simulink model "CubeSat"  (R2024b)
settings: Solver=VariableStepAuto  StartTime=0.0  StopTime=10.0  RelTol=1e-3
undefined symbols (not defined in the file or in its folder): act, env, flag, IC, orb, sat, sens
libraries: matrix_library x14, simulink_extras x2
(part 1 of 3)
settings Model: Creator=filippocamaleonte  LastModifiedBy=filippocamaleonte

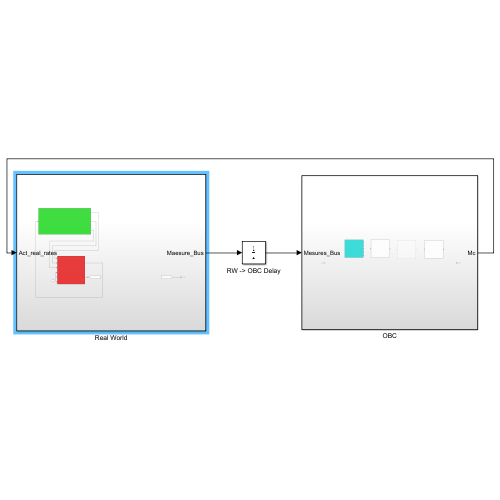
[thumbnail: Simulink's stored preview of the top-level diagram]
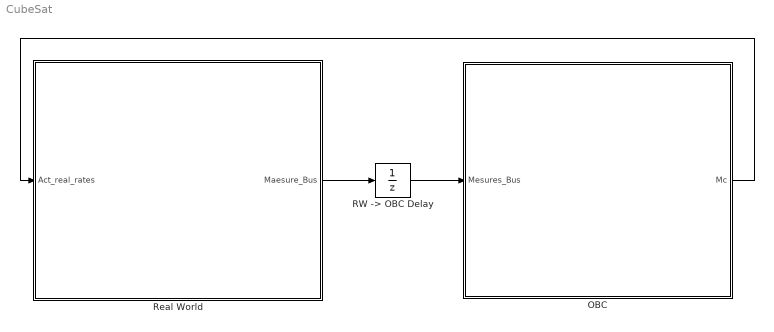
== system CubeSat ==
  OBC : Subsystem
  "RW -> OBC Delay" : UnitDelay  SampleTime=-1  HasFrameUpgradeWarning=on
  Real World : Subsystem
  wires:
  OBC/1(Mc) -> Real World/1(Act_real_rates)
  "RW -> OBC Delay"/1 -> OBC/1(Mesures_Bus)
  Real World/1(Maesure_Bus) -> "RW -> OBC Delay"/1

== system CubeSat/OBC ==
  Mesures_Bus : Inport
  Control : Subsystem
  Guidance : Subsystem
  Navigation : Subsystem  Commented=on
  Reference : Subsystem
  Mc : Outport

== system CubeSat/Real World ==
  Act_real_rates : Inport
  DKE (Dynamics Kinematics Environment) : Subsystem
  Hardware Models : Subsystem
  Maesure_Bus : Outport
  wires:
  Hardware Models/1(Control_Torque_Real) -> DKE (Dynamics Kinematics Environment)/1(M_control)
  DKE (Dynamics Kinematics Environment)/3(Eclipse) -> Hardware Models/3(Eclipse)
  DKE (Dynamics Kinematics Environment)/1(w_b) -> Hardware Models/1(w_b)
  DKE (Dynamics Kinematics Environment)/2(s_b) -> Hardware Models/2(S_b)
  Act_real_rates/1 -> Hardware Models/4(Mc_b)
  Hardware Models/2(Measure_Bus) -> [Measure_Bus]
  [Measure_Bus] -> Maesure_Bus/1

== system CubeSat/OBC/Control ==
  In1 : Inport
  Out1 : Outport
  wires:
  In1/1 -> Out1/1

== system CubeSat/OBC/Guidance ==
  In1 : Inport
  Out1 : Outport
  wires:
  In1/1 -> Out1/1

== system CubeSat/OBC/Navigation ==
  In1 : Inport
  Subsystem1 : Subsystem
  Out1 : Outport

== system CubeSat/OBC/Reference ==
  Conical Shadow Model : Subsystem
  Constant1 : Constant  Value=orb.i
  Kepler Integrator Ref : Subsystem
  LVLH Evolution wtr of Earth : Subsystem
  Magnetic Field order 1 : Subsystem
  SpaceCraft position wrt ECI : Subsystem
  Sun Direction Circular Orbit : Subsystem
  A_ln : Outport
  r_n : Outport  Port=2
  S_n : Outport  Port=3
  eclipseFlag : Outport  Port=4
  B_n : Outport  Port=5
  wires:
  Kepler Integrator Ref/1(th_ref) -> SpaceCraft position wrt ECI/1(th), LVLH Evolution wtr of Earth/1(th)
  Constant1/1 -> LVLH Evolution wtr of Earth/2(i)
  LVLH Evolution wtr of Earth/1(A_ln) -> A_ln/1
  Sun Direction Circular Orbit/1(S_n) -> S_n/1, Conical Shadow Model/1(S_n)
  SpaceCraft position wrt ECI/1(r_n) -> Magnetic Field order 1/1(Vector), r_n/1, Conical Shadow Model/2(r_n)
  Conical Shadow Model/1(eclipseFlag) -> eclipseFlag/1
  Magnetic Field order 1/1(B_n) -> B_n/1

== system CubeSat/Real World/DKE (Dynamics Kinematics Environment) ==
  M_control : Inport
  Dynamics : Subsystem
  Environment : Subsystem
  Kinematics : Subsystem
  Sum : Sum  Inputs=|++
  w_b : Outport
  s_b : Outport  Port=2
  Eclipse : Outport  Port=3
  wires:
  M_control/1 -> Sum/1
  Dynamics/1(w_b) -> [w_b], Kinematics/1(w_b)
  Sum/1 -> Dynamics/1(M_ext)
  Environment/3(Disturbance_torque) -> Sum/2
  [w_b] -> w_b/1
  Environment/1(Eclipse) -> Eclipse/1
  Kinematics/3(r_n) -> Environment/3(r_n)
  Kinematics/1(A_bn) -> Environment/1(A_bn)
  Kinematics/2(A_bl) -> Environment/2(A_bl)

== system CubeSat/Real World/Hardware Models ==
  note: Hardware Models
  note: Input Interface
  note: Output Interface
  w_b : Inport
  S_b : Inport  Port=2
  Eclipse : Inport  Port=3
  Mc_b : Inport  Port=4
  B_b : Inport  Port=5
  w_est_b : Inport  Port=6
  Actuators : Subsystem
  Sensors : Subsystem
  Control_Torque_Real : Outport
  Measure_Bus : Outport  Port=2
  wires:
  Sensors/1(Measure) -> [measure_bus]
  [measure_bus] -> Measure_Bus/1
  [S_b] -> Sensors/1(S_b)
  [control_torque] -> Control_Torque_Real/1
  Actuators/1(Control_Torque_b) -> [control_torque]
  [eclipse] -> Sensors/2(Eclipse)
  S_b/1 -> [S_b]
  Eclipse/1 -> [eclipse]
  B_b/1 -> [B_b]
  w_est_b/1 -> [w_est_b]
  w_b/1 -> [w_b]
  Mc_b/1 -> [Mc_b]
  [B_b] -> Sensors/3(B_b)
  [w_est_b] -> Actuators/2(w_est_b)
  [w_b] -> Actuators/3(w_b)
  [Mc_b] -> Actuators/1(Mc_b)

== system CubeSat/OBC/Navigation/Subsystem1 ==
  S_b : Inport
  S_N : Inport  Port=2
  B_b : Inport  Port=3
  B_N : Inport  Port=4
  alpha 1 : Inport  Port=5
  alpha 2 : Inport  Port=6
  B computing : Subsystem
      settings: PortSchema="{\"entries\":[{\"content\":{\"sides\":[{\"content\":{\"connectorIds\":[\"In1\",\"In2\",\"In3\",\"In4\"]},\"type\":\"ConnectorPlacement.EquallySpacedRectSide\",\"uuid\":\"50fc9399-82b5-4b10-921b-f93011029ce3\"},{\"content\":{\"connectorIds\":[\"Out1\"],\"side\":\"RIGHT\"},\"type\":\"ConnectorPlacement.EquallySpacedRectSide\",\"uuid\":\"3981c554-ab38-4f62-9b84-94877d1cd2ff\"},{\"content\":{\"connectorIds\":[\"In5\",\"In6\"],\"side\":\"TOP\"},\"type\":\"ConnectorPlacement.EquallySpacedRectSide\",\"uuid\":\"ba062d99-6f44-4068-8114-c0cfa81f1ff2\"},{\"content\":{\"side\":\"BOTTOM\"},\"type\":\"ConnectorPlacement.EquallySpacedRectSide\",\"uuid\":\"0ce0d8e8-da8b-4b2d-90df-7b0bc851bc5b\"}]},\"type\":\"ConnectorPlacement.EquallySpacedConnector\",\"uuid\":\"bcda7430-c6c8-4f59-a99a-b367d20ffcb5\"}],\"packageUris\":[\"http://schema.mathworks.com/mf0/Connector/R2020b\"],\"version\":\"1.0\"}"
  Constant : Constant  Value=0
  K matrix computing : Subsystem
  MAGNETOMETER : Subsystem
  Subsystem : Subsystem
      settings: PortSchema="{\"entries\":[{\"content\":{\"sides\":[{\"content\":{\"connectorIds\":[\"In1\",\"In2\"]},\"type\":\"ConnectorPlacement.EquallySpacedRectSide\",\"uuid\":\"5768cb62-7f28-4cce-8da1-dcdd14add895\"},{\"content\":{\"connectorIds\":[\"Out1\"],\"side\":\"RIGHT\"},\"type\":\"ConnectorPlacement.EquallySpacedRectSide\",\"uuid\":\"8778aa17-5802-4f6c-9df9-b85455c7c074\"},{\"content\":{\"connectorIds\":[\"In3\",\"In4\",\"In5\"],\"side\":\"TOP\"},\"type\":\"ConnectorPlacement.EquallySpacedRectSide\",\"uuid\":\"8a3cb844-269f-4d3f-b8ee-2af4584390c1\"},{\"content\":{\"connectorIds\":[\"In6\",\"In7\",\"In8\",\"In9\"],\"side\":\"BOTTOM\"},\"type\":\"ConnectorPlacement.EquallySpacedRectSide\",\"uuid\":\"ccc3bad4-265e-44f4-a8b0-aae769a28e60\"}]},\"type\":\"ConnectorPlacement.EquallySpacedConnector\",\"uuid\":\"9389ccda-4d08-49a8-9951-bd9019203c57\"}],\"packageUris\":[\"http://schema.mathworks.com/mf0/Connector/R2020b\"],\"version\":\"1.0\"}"
  Sun Sensor (S0) : Subsystem
  quaternion to DCM : Subsystem
  DCM : Outport
  wires:
  alpha 1/1 -> Subsystem/5(alpha1), B computing/5(alpha 1)
  S_b/1 -> [S_b]
  [B_N] -> Subsystem/7(B_N)
  Sun Sensor (S0)/1(S_mes_b) -> B computing/1(Sb)
  Constant/1 -> Sun Sensor (S0)/2(eclipse)
  B_b/1 -> [B_b]
  MAGNETOMETER/1(B_meas) -> B computing/3(Bb)
  alpha 2/1 -> B computing/6(alpha 2), Subsystem/4(alpha2)
  [B_N] -> B computing/4(BN)
  [B_b] -> Subsystem/6(B_b)
  [S_b] -> Subsystem/8(S_b)
  [S_N] -> B computing/2(SN)
  S_N/1 -> [S_N]
  [S_b] -> Sun Sensor (S0)/1(S_b)
  B_N/1 -> [B_N]
  B computing/1(B) -> Subsystem/3(B), K matrix computing/1(B)
  K matrix computing/2(Z) -> Subsystem/2(Z)
  quaternion to DCM/1(DCM) -> DCM/1
  K matrix computing/1(S) -> Subsystem/1(S)
  [S_N] -> Subsystem/9(S_N)
  [B_b] -> MAGNETOMETER/1(B_real)
  Subsystem/1(q_opt) -> quaternion to DCM/1(q_opt)

== system CubeSat/OBC/Reference/Conical Shadow Model ==
  note: Output Interface
  note: Input Interface
  note: Model is cylindrical shadow, formula was taken by Crassidis
  S_n : Inport
  r_n : Inport  Port=2
  Dot Product : DotProduct  OutDataTypeStr=Inherit: Inherit via internal rule
  Earth's Radius : Constant  Value=env.Earth.R
  Eclipse (1) : Subsystem  TreatAsAtomicUnit=on
  Gain : Gain  Gain=-1
  If : If  NumInputs=2  IfExpression=u1 < u2
  Merge : Merge
  Norm : Subsystem
  NotEclipse (0) : Subsystem  TreatAsAtomicUnit=on
  Sqrt : Sqrt
  Square : Math  Operator=square
  Square1 : Math  Operator=square
  Subtract : Sum  Inputs=+-
  eclipseFlag : Outport
  wires:
  r_n/1 -> Dot Product/2, Norm/1(Vector)  "r_n"
  S_n/1 -> Dot Product/1  "S_n"
  Norm/1(Norm) -> Square1/1  "norm_r"
  If/1 -> Eclipse (1)/Action
  If/2 -> NotEclipse (0)/Action
  Merge/1 -> eclipseFlag/1
  Eclipse (1)/1(One) -> Merge/1
  NotEclipse (0)/1(Zero) -> Merge/2
  Dot Product/1 -> If/1
  Gain/1 -> If/2
  Sqrt/1 -> Gain/1
  Subtract/1 -> Sqrt/1
  Square/1 -> Subtract/2
  Square1/1 -> Subtract/1
  Earth's Radius/1 -> Square/1  "earth_R"

== system CubeSat/OBC/Reference/Kepler Integrator Ref ==
  Add : Sum  Inputs=+-
  Add1 : Sum
  Constant : Constant  Value=IC.theta
  Constant1 : Constant  Value=3/2
  Constant2 : Constant
  Constant3 : Constant  Value=2
  Constant4 : Constant  Value=orb.e
  Constant5 : Constant  Value=2
  Constant6 : Constant
  Cosh : Trigonometry  Operator=cos
  Divide : Product  Inputs=*/
  Gain : Gain  Gain=orb.n
  Gain1 : Gain  Gain=orb.e
  Integrator : Integrator  InitialConditionSource=external  WrapState=on  WrappedStateUpperValue=2*pi  WrappedStateLowerValue=0
  Power : Math  Operator=pow
  Power1 : Math  Operator=pow
  Power2 : Math  Operator=pow
  th_ref : Outport
  wires:
  Constant/1 -> Integrator/2
  Integrator/1 -> Cosh/1, th_ref/1
  Divide/1 -> Integrator/1
  Power/1 -> Divide/2
  Constant1/1 -> Power/2
  Constant2/1 -> Add/1
  Add/1 -> Power/1
  Power1/1 -> Add/2
  Constant3/1 -> Power1/2
  Constant4/1 -> Power1/1
  Gain/1 -> Divide/1
  Power2/1 -> Gain/1
  Constant5/1 -> Power2/2
  Add1/1 -> Power2/1
  Constant6/1 -> Add1/1
  Gain1/1 -> Add1/2
  Cosh/1 -> Gain1/1

== system CubeSat/OBC/Reference/LVLH Evolution wtr of Earth ==
  th : Inport
  i : Inport  Port=2
  Constant1 : Constant
  Constant{2,4..10} (8 alike) : Constant  Value=0
  Constant3 : Constant
  Cos : Trigonometry  Operator=cos
  Cos1 : Trigonometry  Operator=cos
  Gain : Gain  Gain=-1
  Gain1 : Gain  Gain=-1
  Matrix Concatenate{,1..2,4..6} (6 alike) : Concatenate  NumInputs=3  Mode=Multidimensional array
  Matrix Concatenate3 : Concatenate  NumInputs=3  Mode=Multidimensional array  ConcatenateDimension=2
  Matrix Concatenate7 : Concatenate  NumInputs=3  Mode=Multidimensional array  ConcatenateDimension=2
  Matrix Multiply : Product  Multiplication=Matrix(*)
  Sin : Trigonometry
  Sin1 : Trigonometry
  A_ln : Outport
  wires:
  Cos/1 -> [cos]
  Matrix Concatenate1/1 -> Matrix Concatenate3/3
  th/1 -> Cos/1, Sin/1
  Matrix Concatenate/1 -> Matrix Concatenate3/1
  Constant5/1 -> Matrix Concatenate1/1
  Constant3/1 -> Matrix Concatenate1/3
  [cos] -> Matrix Concatenate/1
  Sin/1 -> [sin]
  Constant6/1 -> Matrix Concatenate2/3
  Constant7/1 -> Matrix Concatenate/3
  Constant4/1 -> Matrix Concatenate1/2
  Matrix Concatenate2/1 -> Matrix Concatenate3/2
  [cos] -> Matrix Concatenate2/2
  [sin] -> Matrix Concatenate2/1
  Gain/1 -> Matrix Concatenate/2
  [sin] -> Gain/1
  Cos1/1 -> [cosi]
  Sin1/1 -> [sini]
  i/1 -> Cos1/1, Sin1/1
  Matrix Multiply/1 -> A_ln/1
  Matrix Concatenate3/1 -> Matrix Multiply/1
  Matrix Concatenate7/1 -> Matrix Multiply/2
  Matrix Concatenate6/1 -> Matrix Concatenate7/2
  Matrix Concatenate5/1 -> Matrix Concatenate7/3
  Matrix Concatenate4/1 -> Matrix Concatenate7/1
  Constant1/1 -> Matrix Concatenate4/1
  Constant2/1 -> Matrix Concatenate4/2
  Constant8/1 -> Matrix Concatenate4/3
  Constant9/1 -> Matrix Concatenate6/1
  Constant10/1 -> Matrix Concatenate5/1
  [cosi] -> Matrix Concatenate5/3
  [cosi] -> Matrix Concatenate6/2
  [sini] -> Matrix Concatenate5/2
  [sini] -> Gain1/1
  Gain1/1 -> Matrix Concatenate6/3

== system CubeSat/OBC/Reference/Magnetic Field order 1 ==
  Vector : Inport
  Clock : Clock
  Constant : Constant  Value=env.mag.dgrf2020
  Constant1 : Constant  Value=env.Earth.R
  Constant2 : Constant  Value=3
  Constant3 : Constant  Value=env.Earth.magInclination
  Constant4 : Constant  Value=3
  Cos : Trigonometry  Operator=cos
  Cos1 : Trigonometry  Operator=cos
  Divide : Product  Inputs=***/
  Divide1 : Product  Inputs=*/
  Divide2 : Product  Inputs=*/
  Dot Product : DotProduct  OutDataTypeStr=Inherit: Inherit via internal rule
  Gain : Gain  Gain=3
  Gain1 : Gain  Gain=env.Earth.omega
  Mux : Mux  Inputs=3
  Norm : Subsystem
  Norm1 : Subsystem
  Norm2 : Subsystem
  Power : Math  Operator=pow
  Power1 : Math  Operator=pow
  Product : Product
  Product1 : Product
  Product2 : Product
  Sin : Trigonometry
  Sin1 : Trigonometry
  Sqrt : Sqrt
  Square : Math  Operator=square
  Subtract : Sum  Inputs=+-
  Sum of Elements : Sum  Inputs=+
  B_n : Outport
  wires:
  Constant/1 -> Square/1
  Square/1 -> Sum of Elements/1
  Sum of Elements/1 -> Sqrt/1
  Constant1/1 -> Power/1
  Constant2/1 -> Power/2
  Sqrt/1 -> Divide/2
  Power/1 -> Divide/3
  Constant4/1 -> Power1/2
  Power1/1 -> Divide/4
  Norm/1(Norm) -> Power1/1  "norm_r"
  Vector/1 -> Norm2/1(Vector), Divide2/1, [rr]
  [rr] -> Norm/1(Vector)
  [rr_hat] -> Dot Product/2
  Subtract/1 -> Divide/1
  [mm] -> Subtract/2
  Dot Product/1 -> Product/2
  Product/1 -> Gain/1
  Gain/1 -> Subtract/1
  [rr_hat] -> Product/1
  [mm] -> Dot Product/1
  Mux/1 -> Norm1/1(Vector), Divide1/1
  Cos/1 -> Mux/3
  Constant3/1 -> Sin/1, Cos/1
  Clock/1 -> Gain1/1
  Sin/1 -> Product2/2, Product1/2
  Product1/1 -> Mux/2
  Product2/1 -> Mux/1
  Cos1/1 -> Product2/1
  Gain1/1 -> Cos1/1, Sin1/1
  Sin1/1 -> Product1/1
  Divide/1 -> B_n/1
  Norm1/1(Norm) -> Divide1/2  "norm_r"
  Divide1/1 -> [mm]
  Norm2/1(Norm) -> Divide2/2  "norm_r"
  Divide2/1 -> [rr_hat]

== system CubeSat/OBC/Reference/SpaceCraft position wrt ECI ==
  th : Inport
  Add : Sum
  Add1 : Sum  Inputs=+-
  Constant : Constant  Value=orb.i
  Constant1 : Constant  Value=orb.i
  Constant2 : Constant
  Constant3 : Constant
  Constant4 : Constant  Value=2
  Constant5 : Constant  Value=orb.e
  Cos : Trigonometry  Operator=cos
  Cos1 : Trigonometry  Operator=cos
  Cos2 : Trigonometry  Operator=cos
  Divide : Product  Inputs=*/
  Gain : Gain  Gain=orb.e
  Gain1 : Gain  Gain=orb.a
  Matrix Concatenate : Concatenate  NumInputs=3  Mode=Multidimensional array
  Power : Math  Operator=pow
  Product : Product
  Product1 : Product
  Product2 : Product
  Sin : Trigonometry
  Sin1 : Trigonometry
  r_n : Outport
  wires:
  Constant/1 -> Sin/1
  Cos1/1 -> Matrix Concatenate/1
  th/1 -> Sin1/1, Cos2/1, Cos1/1
  Product1/1 -> Matrix Concatenate/2
  Product/1 -> Matrix Concatenate/3
  Sin1/1 -> Product1/2, Product/1
  Sin/1 -> Product/2
  Constant1/1 -> Cos/1
  Cos/1 -> Product1/1
  Product2/1 -> r_n/1
  Matrix Concatenate/1 -> Product2/1
  Divide/1 -> Product2/2
  Constant2/1 -> Add/1
  Add/1 -> Divide/2
  Cos2/1 -> Gain/1
  Gain/1 -> Add/2
  Constant3/1 -> Add1/1
  Power/1 -> Add1/2
  Constant4/1 -> Power/2
  Constant5/1 -> Power/1
  Add1/1 -> Gain1/1
  Gain1/1 -> Divide/1

== system CubeSat/OBC/Reference/Sun Direction Circular Orbit ==
  note: Input Interface
  note: Output Interface
  Clock : Clock
  Cos : Trigonometry  Operator=cos
  Cos1 : Trigonometry  Operator=cos
  Earth's Inclination : Constant  Value=env.Earth.i
  Gain : Gain  Gain=env.Earth.n
  Matrix Concatenate : Concatenate  NumInputs=3  Mode=Multidimensional array
  Product : Product
  Product1 : Product
  Product2 : Product
  Sin : Trigonometry
  Sin1 : Trigonometry
  Sun's Radius : Constant  Value=env.Sun.R
  S_n : Outport
  wires:
  Clock/1 -> Gain/1
  Gain/1 -> Sin/1, Cos/1
  Product/1 -> S_n/1
  Sun's Radius/1 -> Product/2
  Matrix Concatenate/1 -> Product/1
  Earth's Inclination/1 -> Sin1/1, Cos1/1
  Cos1/1 -> [cos]
  Sin1/1 -> [sin]
  Cos/1 -> Matrix Concatenate/1
  Product1/1 -> Matrix Concatenate/2
  Product2/1 -> Matrix Concatenate/3
  [sin] -> Product2/2
  [cos] -> Product1/1
  Sin/1 -> Product1/2, Product2/1

== system CubeSat/Real World/DKE (Dynamics Kinematics Environment)/Dynamics ==
  note: Here we need both Newton and Euler Law
  M_ext : Inport
  Euler Integrator : Subsystem
  w_b : Outport
  wires:
  M_ext/1 -> Euler Integrator/1(M_ext)
  Euler Integrator/1(w_b) -> w_b/1

== system CubeSat/Real World/DKE (Dynamics Kinematics Environment)/Environment ==
  note: Enviroment Models (Celestial Objects, Shadow, Magnetic Field, atmosphere, albedo)
  A_bn : Inport
  A_bl : Inport  Port=2
  r_n : Inport  Port=3
  Conical Shadow Model : Subsystem
  Perturbations : Subsystem
  Sun Direction Circular Orbit : Subsystem
  Eclipse : Outport
  s_n : Outport  Port=2
  Disturbance_torque : Outport  Port=3
  wires:
  Sun Direction Circular Orbit/1(S_n) -> [S_n], s_n/1, Conical Shadow Model/1(S_n)
  Conical Shadow Model/1(eclipseFlag) -> Eclipse/1
  Perturbations/1(Disturbance_torque) -> Disturbance_torque/1
  r_n/1 -> Perturbations/2(r_n), Conical Shadow Model/2(r_n)
  A_bn/1 -> Perturbations/3(A_bn)
  [S_n] -> Perturbations/1(S_n)  "S_n"
  A_bl/1 -> Perturbations/4(A_bl)

== system CubeSat/Real World/DKE (Dynamics Kinematics Environment)/Kinematics ==
  note: B/N calculation
      | Keplerian calculations
      | L/N calculation
      | B/L calculation
  w_b : Inport
  Attitude Error : Subsystem
  Constant1 : Constant  Value=orb.i
  EulerKinematicsdelay : Subsystem
  Kepler Integrator1 : Subsystem
  LVLH Evolution wtr of Earth : Subsystem
  SpaceCraft position wrt ECI : Subsystem
  A_bn : Outport
  A_bl : Outport  Port=2
  r_n : Outport  Port=3
  wires:
  w_b/1 -> EulerKinematicsdelay/1(w_b)
  Attitude Error/1(A_bl) -> A_bl/1
  EulerKinematicsdelay/1(A_bn) -> A_bn/1, Attitude Error/1(A_bn)
  LVLH Evolution wtr of Earth/1(A_ln) -> Attitude Error/2(A_ln)
  Constant1/1 -> LVLH Evolution wtr of Earth/2(i)
  Kepler Integrator1/1(th) -> SpaceCraft position wrt ECI/1(th), LVLH Evolution wtr of Earth/1(th)
  SpaceCraft position wrt ECI/1(r_n) -> r_n/1

== system CubeSat/Real World/Hardware Models/Actuators ==
  Mc_b : Inport
  w_est_b : Inport  Port=2
  w_b : Inport  Port=3
  CMG + Control Logic : Subsystem
  Control_Torque_b : Outport

== system CubeSat/Real World/Hardware Models/Sensors ==
  note: Sun direction versor, MUST be normalised outside
  note: Input Interface
  note: Sun Sensors Array
  note: Output Interface
  note: Magnetometer
  S_b : Inport
  Eclipse : Inport  Port=2
  B_b : Inport  Port=3
  Bus Creator : BusCreator  Inputs=2
  MAGNETOMETER : Subsystem
  SS Selector : Subsystem
  Sun Sensor (Fine) : Subsystem
  Sun Sensor (S1) : Subsystem
  Sun Sensor (S2) : Subsystem
  Sun Sensor (S3) : Subsystem
  Sun Sensor (S4) : Subsystem
  Measure : Outport
  wires:
  Sun Sensor (S3)/1(S_meas_b) -> SS Selector/4(Course SS 3)
  Sun Sensor (Fine)/1(S_meas_b) -> SS Selector/1(Fine SS)
  Sun Sensor (S4)/1(S_meas_b) -> SS Selector/5(Course SS 4)
  Sun Sensor (S1)/1(S_meas_b) -> SS Selector/2(Course SS 1)
  Sun Sensor (S2)/1(S_meas_b) -> SS Selector/3(Course SS 2)
  S_b/1 -> [S_b]
  [S_b] -> Sun Sensor (S1)/1(S_b)
  [S_b] -> Sun Sensor (Fine)/1(S_b)
  [S_b] -> Sun Sensor (S2)/1(S_b)
  [S_b] -> Sun Sensor (S3)/1(S_b)
  [S_b] -> Sun Sensor (S4)/1(S_b)
  Eclipse/1 -> [eclipse]
  [eclipse] -> Sun Sensor (Fine)/2(eclipse)
  [eclipse] -> Sun Sensor (S1)/2(eclipse)
  [eclipse] -> Sun Sensor (S2)/2(eclipse)
  [eclipse] -> Sun Sensor (S3)/2(eclipse)
  [eclipse] -> Sun Sensor (S4)/2(eclipse)
  SS Selector/1(S_meas_b) -> [S_meas_b]
  Bus Creator/1 -> Measure/1  "Measure_bus"
  [S_meas_b] -> Bus Creator/1  "S_meas_b"
  [B_meas_b] -> Bus Creator/2  "B_meas_b"
  MAGNETOMETER/1(B_meas_b) -> [B_meas_b]
  B_b/1 -> [B_b]
  [B_b] -> MAGNETOMETER/1(B_b)

== system CubeSat/OBC/Navigation/Subsystem1/B computing ==
  Sb : Inport
  SN : Inport  Port=2
  Bb : Inport  Port=3
  BN : Inport  Port=4
  alpha 1 : Inport  Port=5
  alpha 2 : Inport  Port=6
  Add : Sum
  Add1 : Sum
  Add2 : Sum
  Divide : Product  Inputs=*/
  Divide1 : Product  Inputs=/*
  Product : Product  Inputs=3  Multiplication=Matrix(*)
  Product1 : Product  Inputs=3  Multiplication=Matrix(*)
  Transpose : Math  Operator=transpose
  Transpose1 : Math  Operator=transpose
  B : Outport
  wires:
  alpha 1/1 -> [alpha_1]
  alpha 2/1 -> [alpha_2]
  [alpha_1] -> Divide/1, Add/1
  [alpha_2] -> Add/2
  Add/1 -> Divide/2
  Divide/1 -> [alpha_1_normalised]
  [alpha_2] -> Divide1/2, Add1/2
  Divide1/1 -> [alpha_2_normalised]
  [alpha_1] -> Add1/1
  Add1/1 -> Divide1/1
  SN/1 -> [SN]
  Sb/1 -> [Sb]
  Bb/1 -> [Bb]
  BN/1 -> [BN]
  Product/1 -> Add2/1
  Product1/1 -> Add2/2
  [alpha_1_normalised] -> Product/1
  [alpha_2_normalised] -> Product1/1
  [Sb] -> Product/2
  Transpose/1 -> Product/3
  Transpose1/1 -> Product1/3
  [SN] -> Transpose/1
  [Bb] -> Product1/2
  [BN] -> Transpose1/1
  Add2/1 -> B/1

== system CubeSat/OBC/Navigation/Subsystem1/K matrix computing ==
  B : Inport
  Add : Sum
  Add{1..4} (4 alike) : Sum  Inputs=+-
  IdentityMatrix : IdentityMatrix
  Matrix Concatenate : Concatenate  NumInputs=4  Mode=Multidimensional array  ConcatenateDimension=2
  Mux : Mux  Inputs=3
  Product : Product
  Selector : Selector  NumberOfDimensions=2  InputPortWidth=3  IndexOptions=Index vector (dialog),Index vector (dialog)  Indices=2,3  OutputSizes=1,1
  Selector1 : Selector  NumberOfDimensions=2  InputPortWidth=3  IndexOptions=Index vector (dialog),Index vector (dialog)  Indices=3,2  OutputSizes=1,1
  Selector2 : Selector  NumberOfDimensions=2  InputPortWidth=3  IndexOptions=Index vector (dialog),Index vector (dialog)  Indices=3,1  OutputSizes=1,1
  Selector3 : Selector  NumberOfDimensions=2  InputPortWidth=3  IndexOptions=Index vector (dialog),Index vector (dialog)  Indices=1,3  OutputSizes=1,1
  Selector4 : Selector  NumberOfDimensions=2  InputPortWidth=3  IndexOptions=Index vector (dialog),Index vector (dialog)  Indices=1,2  OutputSizes=1,1
  Selector5 : Selector  NumberOfDimensions=2  InputPortWidth=3  IndexOptions=Index vector (dialog),Index vector (dialog)  Indices=2,1  OutputSizes=1,1
  Trace : Subsystem
  Transpose : matrix_library/Transpose
  Transpose1 : matrix_library/Transpose
  S : Outport
  Z : Outport  Port=2
  wires:
  [B] -> Add/1, Transpose/1
  Transpose/1 -> Add/2
  Add/1 -> [S]
  B/1 -> [B]
  [B] -> Trace/1(In1)
  Trace/1(Out1) -> [Sigma]
  [B] -> Selector/1, Selector1/1, Selector2/1, Selector5/1, Selector4/1, Selector3/1
  Selector/1 -> Add1/1
  Selector1/1 -> Add1/2
  Selector4/1 -> Add3/1
  Selector5/1 -> Add3/2
  Selector3/1 -> Add2/2
  Selector2/1 -> Add2/1
  Add1/1 -> Mux/1
  Add2/1 -> Mux/2
  Add3/1 -> Mux/3
  Mux/1 -> [Z]
  [Z] -> Matrix Concatenate/2
  [Sigma] -> Product/1
  IdentityMatrix/1 -> Product/2
  Product/1 -> Add4/2
  [S] -> Add4/1
  Add4/1 -> Matrix Concatenate/1
  Transpose1/1 -> Matrix Concatenate/3
  [Z] -> Transpose1/1
  [Sigma] -> Matrix Concatenate/4
  [S] -> S/1
  [Z] -> Z/1

== system CubeSat/OBC/Navigation/Subsystem1/MAGNETOMETER ==
  note: Also the noise is really low (doesn't appear in the output). Now the noise changes based on the input signal, we can put a fixed value equal to the maximum possible noise (associated to the biggest input)
  note: Need to separate the three components
  note: Missing errors:
      | -SCALE FACTORS ERROR, we can add it to have a more refined model
  B_real : Inport
  Add : Sum
  Cast To Single : DataTypeConversion  OutDataTypeStr=single  SaturateOnIntegerOverflow=off  RndMeth=Floor
  Constant : Constant  Value=sens.mag.flag
  Constant1 : Constant  Value=sens.mag.A_nonorth
  Constant3 : Constant  Value=sens.mag.A_mis
  Matrix Multiply : Product  Multiplication=Matrix(*)
  MatrixMultiply : Product  Multiplication=Matrix(*)
  Noise x : Subsystem
  Switch : Switch  Criteria=u2 > Threshold  SaturateOnIntegerOverflow=off  InputSameDT=off
  "discretization " : ZeroOrderHold  SampleTime=sens.mag.Ts
  quantization : Quantizer  QuantizationInterval=sens.mag.Quant
  saruration : Saturate  UpperLimit=sens.mag.sat(1,1)  LowerLimit=sens.mag.sat(1,2)
  B_meas : Outport
  wires:
  B_real/1 -> [B], Noise x/1(B_real), Matrix Multiply/2
  [B] -> Switch/3
  Constant/1 -> Switch/2
  Switch/1 -> quantization/1
  "discretization "/1 -> Cast To Single/1
  saruration/1 -> "discretization "/1
  quantization/1 -> saruration/1
  Constant3/1 -> Matrix Multiply/1
  Matrix Multiply/1 -> MatrixMultiply/2
  Constant1/1 -> MatrixMultiply/1
  MatrixMultiply/1 -> Add/1
  Cast To Single/1 -> B_meas/1
  Add/1 -> Switch/1
  Noise x/1(Out1) -> Add/2

== system CubeSat/OBC/Navigation/Subsystem1/Subsystem ==
  S : Inport
  Z : Inport  Port=2
  B : Inport  Port=3
  alpha2 : Inport  Port=4
  alpha1 : Inport  Port=5
  B_b : Inport  Port=6
  B_N : Inport  Port=7
  S_b : Inport  Port=8
  S_N : Inport  Port=9
  Add : Sum
  Math Function : Math  Operator=square
  Math Function1 : Math  Operator=square
  q_opt : Outport
  wires:
  alpha2/1 -> Math Function/1
  alpha1/1 -> Math Function1/1
  Math Function/1 -> Add/1
  Math Function1/1 -> Add/2

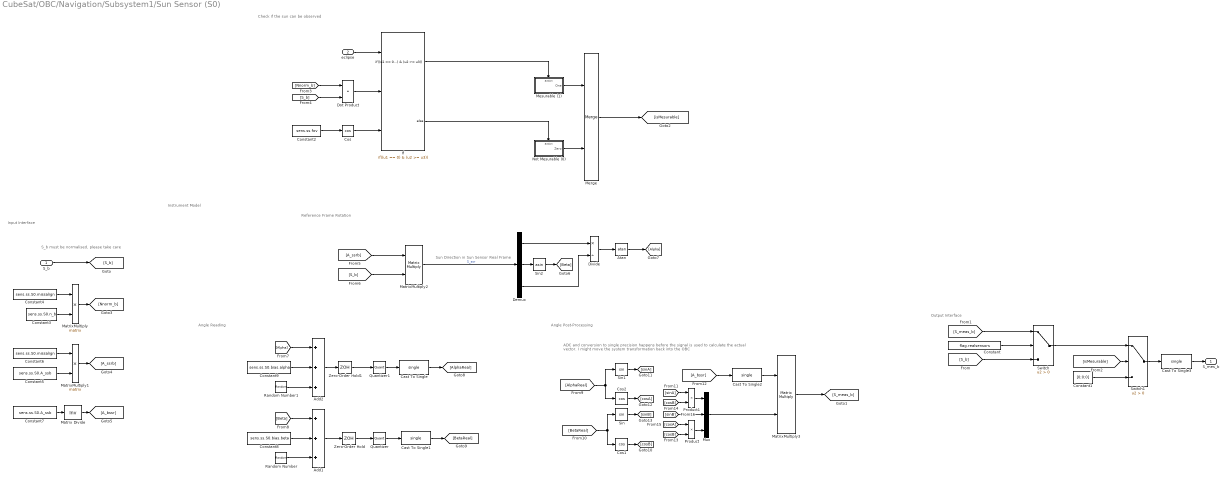
== system CubeSat/OBC/Navigation/Subsystem1/Sun Sensor (S0) ==
  note: Instrument Model
  note: Angle Reading
  note: Reference Frame Rotation
  note: ADC and conversion to single precision happens before the signal is used to calculate the actual vector. I might move the system transformation back into the OBC
  note: Sun Direction in Sun Sensor Real Frame
  note: S_b must be normalised, please take care
  note: Input Interface
  note: Output Interface
  note: Check if the sun can be observed
  note: Angle Post-Processing
  S_b : Inport
  eclipse : Inport  Port=2
  Add1 : Sum  Inputs=+++
  Add2 : Sum  Inputs=+++
  Atan : Trigonometry  Operator=atan
  Cast To Single{,1..3} (4 alike) : DataTypeConversion  OutDataTypeStr=single  SaturateOnIntegerOverflow=off  RndMeth=Floor
  Constant : Constant  Value=flag.realsensors
  Constant1 : Constant  Value=[0;0;0]
  Constant2 : Constant  Value=sens.ss.fov
  Constant3 : Constant  Value=sens.ss.S0.n_b
  Constant4 : Constant  Value=sens.ss.S0.missalign
  Constant5 : Constant  Value=sens.ss.S0.A_ssb
  Constant6 : Constant  Value=sens.ss.S0.missalign
  Constant7 : Constant  Value=sens.ss.S0.A_ssb
  Constant8 : Constant  Value=sens.ss.S0.bias.beta
  Constant9 : Constant  Value=sens.ss.S0.bias.alpha
  Cos : Trigonometry  Operator=cos
  Cos1 : Trigonometry  Operator=cos
  Cos2 : Trigonometry  Operator=cos
  Demux : Demux  Outputs=3
  Divide : Product  Inputs=*/
  Dot Product : DotProduct  OutDataTypeStr=Inherit: Inherit via internal rule
  If : If  NumInputs=3  IfExpression=(u1 == 0) & (u2 >= u3)
  Matrix Divide : Product  Inputs=/  Multiplication=Matrix(*)
  MatrixMultiply{,1..3} (4 alike) : Product  Multiplication=Matrix(*)
  Merge : Merge
  Mesurable (1) : Subsystem  TreatAsAtomicUnit=on
  Mux : Mux  Inputs=3
  Not Mesurable (0) : Subsystem  TreatAsAtomicUnit=on
  Product : Product
  Product1 : Product
  Quantizer : Quantizer  QuantizationInterval=sens.ss.ADC.quanta
  Quantizer1 : Quantizer  QuantizationInterval=sens.ss.ADC.quanta
  Random Number : RandomNumber  Variance=(sens.ss.precision/1.4)^2  Seed=sens.ss.S0.seed.beta  SampleTime=sens.ss.freq
  Random Number1 : RandomNumber  Variance=(sens.ss.precision/1.4)^2  Seed=sens.ss.S0.seed.beta  SampleTime=sens.ss.freq
  Sin : Trigonometry
  Sin1 : Trigonometry
  Sin2 : Trigonometry  Operator=asin
  Switch : Switch  Criteria=u2 > Threshold  SaturateOnIntegerOverflow=off  InputSameDT=off
  Switch1 : Switch  Criteria=u2 > Threshold  SaturateOnIntegerOverflow=off  InputSameDT=off
  Zero-Order Hold : ZeroOrderHold  SampleTime=sens.ss.freq
  Zero-Order Hold1 : ZeroOrderHold  SampleTime=sens.ss.freq
  S_mes_b : Outport
  wires:
  Constant/1 -> Switch/2
  S_b/1 -> [S_b]
  [S_b] -> Switch/3
  [S_meas_b] -> Switch/1
  eclipse/1 -> If/1
  If/1 -> Mesurable (1)/Action
  If/2 -> Not Mesurable (0)/Action
  Not Mesurable (0)/1(Zero) -> Merge/2
  Mesurable (1)/1(One) -> Merge/1
  Cos/1 -> If/3
  Constant2/1 -> Cos/1
  Dot Product/1 -> If/2
  Merge/1 -> [isMesurable]
  [isMesurable] -> Switch1/2
  [Nnorm_b] -> Dot Product/1
  [S_b] -> Dot Product/2
  Switch1/1 -> Cast To Single3/1
  Constant4/1 -> MatrixMultiply/1
  MatrixMultiply/1 -> [Nnorm_b]
  Constant3/1 -> MatrixMultiply/2
  Constant1/1 -> Switch1/3
  Switch/1 -> Switch1/1
  Constant6/1 -> MatrixMultiply1/1
  Constant5/1 -> MatrixMultiply1/2
  MatrixMultiply1/1 -> [A_ssrb]
  Constant7/1 -> Matrix Divide/1
  Matrix Divide/1 -> [A_bssr]
  [A_ssrb] -> MatrixMultiply2/1
  [S_b] -> MatrixMultiply2/2
  MatrixMultiply2/1 -> Demux/1  "S_ssr"
  Demux/1 -> Divide/1
  Demux/3 -> Divide/2
  Sin2/1 -> [Beta]
  Divide/1 -> Atan/1
  Add2/1 -> Zero-Order Hold1/1
  Add1/1 -> Zero-Order Hold/1
  Quantizer1/1 -> Cast To Single/1
  Zero-Order Hold1/1 -> Quantizer1/1
  Quantizer/1 -> Cast To Single1/1
  Zero-Order Hold/1 -> Quantizer/1
  [Alpha] -> Add2/1
  [Beta] -> Add1/1
  Constant8/1 -> Add1/2
  Constant9/1 -> Add2/2
  Cast To Single/1 -> [AlphaReal]
  Cast To Single1/1 -> [BetaReal]
  Random Number/1 -> Add1/3
  Random Number1/1 -> Add2/3
  Cast To Single3/1 -> S_mes_b/1
  MatrixMultiply3/1 -> [S_meas_b]
  Mux/1 -> MatrixMultiply3/2
  Cast To Single2/1 -> MatrixMultiply3/1
  [A_bssr] -> Cast To Single2/1
  [BetaReal] -> Cos1/1, Sin/1
  Atan/1 -> [Alpha]
  [AlphaReal] -> Cos2/1, Sin1/1
  Product/1 -> Mux/3
  Product1/1 -> Mux/1
  Demux/2 -> Sin2/1
  Sin1/1 -> [sinA]
  Cos2/1 -> [cosA]
  [sinA] -> Product1/1
  Cos1/1 -> [cosB]
  [cosB] -> Product/2
  [cosB] -> Product1/2
  [cosA] -> Product/1
  Sin/1 -> [sinB]
  [sinB] -> Mux/2

== system CubeSat/OBC/Navigation/Subsystem1/quaternion to DCM ==
  q_opt : Inport
  Add : Sum  Inputs=+-
  Add1 : Sum  Inputs=++-
  Constant : Constant  Value=2
  Constant1 : Constant  Value=0
  Constant2 : Constant  Value=0
  Constant3 : Constant  Value=0
  Constant4 : Constant  Value=-1
  Constant5 : Constant  Value=-1
  Constant6 : Constant  Value=-1
  Constant7 : Constant  Value=2
  IdentityMatrix : IdentityMatrix
  Math Function : Math  Operator=square
  Matrix Concatenate : Concatenate  NumInputs=9  Mode=Multidimensional array  ConcatenateDimension=3
  Product : Product  Multiplication=Matrix(*)
  Product{1..2,5..7} (5 alike) : Product
  Product3 : Product  Multiplication=Matrix(*)
  Product4 : Product  Inputs=3
  Selector1 : Selector  InputPortWidth=4  IndexOptions=Index vector (dialog)  Indices=4  OutputSizes=1
  Selector2 : Selector  InputPortWidth=4  IndexOptions=Index vector (dialog)  Indices=4  OutputSizes=1
  Selector3 : Selector  InputPortWidth=4  IndexOptions=Index vector (dialog)  Indices=2  OutputSizes=1
  Selector4 : Selector  InputPortWidth=4  IndexOptions=Index vector (dialog)  Indices=1  OutputSizes=1
  Transpose : Math  Operator=transpose
  Transpose1 : Math  Operator=transpose
  DCM : Outport
  wires:
  [q4] -> Math Function/1
  Math Function/1 -> Add/1
  Product/1 -> Add/2
  Transpose/1 -> Product/1
  Add/1 -> Product1/1
  IdentityMatrix/1 -> Product1/2
  q_opt/1 -> [q_opt]
  [q_opt] -> Transpose/1, Product/2
  Constant/1 -> Product2/1
  [q_opt] -> Transpose1/1, Product2/2
  Product2/1 -> Product3/1
  Transpose1/1 -> Product3/2
  Product3/1 -> [A2]
  Product1/1 -> [A1]
  [q_opt] -> Selector1/1
  Selector1/1 -> [q4]
  Product4/1 -> [A3]
  Add1/1 -> DCM/1
  [A1] -> Add1/1
  [A2] -> Add1/2
  [A3] -> Add1/3
  [q_opt] -> Selector2/1
  Selector2/1 -> [q3]
  [q_opt] -> Selector3/1
  Selector3/1 -> [q2]
  [q_opt] -> Selector4/1
  Selector4/1 -> [q1]
  Matrix Concatenate/1 -> [q_matrix]
  Constant1/1 -> Matrix Concatenate/1
  Constant2/1 -> Matrix Concatenate/5
  Constant3/1 -> Matrix Concatenate/9
  [q2] -> Matrix Concatenate/3
  [q3] -> Matrix Concatenate/4
  [q1] -> Matrix Concatenate/8
  Product5/1 -> Matrix Concatenate/7
  Product6/1 -> Matrix Concatenate/6
  Product7/1 -> Matrix Concatenate/2
  [q3] -> Product7/1
  Constant4/1 -> Product7/2
  Constant5/1 -> Product6/1
  Constant6/1 -> Product5/2
  [q1] -> Product6/2
  [q2] -> Product5/1
  [q_matrix] -> Product4/3
  [q4] -> Product4/2
  Constant7/1 -> Product4/1

== system CubeSat/OBC/Reference/Conical Shadow Model/Eclipse (1) ==
  Action Port : ActionPort  ActionPortLabel=if(u1 < u2)
  Constant : Constant
  One : Outport
  wires:
  Constant/1 -> One/1

== system CubeSat/OBC/Reference/Conical Shadow Model/Norm ==
  Vector : Inport
  Add : Sum  Inputs=+++
  Demux : Demux  Outputs=3
  Sqrt : Sqrt
  Square : Math  Operator=square
  Square1 : Math  Operator=square
  Square2 : Math  Operator=square
  Norm : Outport
  wires:
  Square/1 -> Add/1
  Add/1 -> Sqrt/1
  Demux/3 -> Square1/1
  Square2/1 -> Add/2
  Square1/1 -> Add/3
  Demux/1 -> Square/1
  Demux/2 -> Square2/1
  Vector/1 -> Demux/1
  Sqrt/1 -> Norm/1

== system CubeSat/OBC/Reference/Conical Shadow Model/NotEclipse (0) ==
  Action Port : ActionPort  ActionPortLabel=else
  Constant : Constant  Value=0
  Zero : Outport
  wires:
  Constant/1 -> Zero/1

== system CubeSat/OBC/Reference/Magnetic Field order 1/Norm ==
  Vector : Inport
  Add : Sum  Inputs=+++
  Demux : Demux  Outputs=3
  Sqrt : Sqrt
  Square : Math  Operator=square
  Square1 : Math  Operator=square
  Square2 : Math  Operator=square
  Norm : Outport
  wires:
  Square/1 -> Add/1
  Add/1 -> Sqrt/1
  Demux/3 -> Square1/1
  Square2/1 -> Add/2
  Square1/1 -> Add/3
  Demux/1 -> Square/1
  Demux/2 -> Square2/1
  Vector/1 -> Demux/1
  Sqrt/1 -> Norm/1

== system CubeSat/OBC/Reference/Magnetic Field order 1/Norm1 ==
  Vector : Inport
  Add : Sum  Inputs=+++
  Demux : Demux  Outputs=3
  Sqrt : Sqrt
  Square : Math  Operator=square
  Square1 : Math  Operator=square
  Square2 : Math  Operator=square
  Norm : Outport
  wires:
  Square/1 -> Add/1
  Add/1 -> Sqrt/1
  Demux/3 -> Square1/1
  Square2/1 -> Add/2
  Square1/1 -> Add/3
  Demux/1 -> Square/1
  Demux/2 -> Square2/1
  Vector/1 -> Demux/1
  Sqrt/1 -> Norm/1

== system CubeSat/OBC/Reference/Magnetic Field order 1/Norm2 ==
  Vector : Inport
  Add : Sum  Inputs=+++
  Demux : Demux  Outputs=3
  Sqrt : Sqrt
  Square : Math  Operator=square
  Square1 : Math  Operator=square
  Square2 : Math  Operator=square
  Norm : Outport
  wires:
  Square/1 -> Add/1
  Add/1 -> Sqrt/1
  Demux/3 -> Square1/1
  Square2/1 -> Add/2
  Square1/1 -> Add/3
  Demux/1 -> Square/1
  Demux/2 -> Square2/1
  Vector/1 -> Demux/1
  Sqrt/1 -> Norm/1

== system CubeSat/Real World/DKE (Dynamics Kinematics Environment)/Dynamics/Euler Integrator ==
  M_ext : Inport
  Constant : Constant  Value=sat.I
  Constant1 : Constant  Value=IC.w0  VectorParams1D=off
  Constant2 : Constant  Value=sat.invI
  Cross Product : matrix_library/Cross Product
  Divide : Product  Inputs=**  Multiplication=Matrix(*)
  Integrator : Integrator  InitialConditionSource=external
  Product : Product  Multiplication=Matrix(*)
  Sum : Sum  Inputs=|++
  w_b : Outport
  wires:
  Product/1 -> Cross Product/1
  Divide/1 -> Integrator/1
  Constant/1 -> Product/1
  Constant2/1 -> Divide/1
  Integrator/1 -> Product/2, Cross Product/2, w_b/1
  Constant1/1 -> Integrator/2
  Cross Product/1 -> Sum/1
  Sum/1 -> Divide/2
  M_ext/1 -> Sum/2

== system CubeSat/Real World/DKE (Dynamics Kinematics Environment)/Environment/Conical Shadow Model ==
  note: Output Interface
  note: Input Interface
  note: Model is cylindrical shadow, formula was taken by Crassidis
  S_n : Inport
  r_n : Inport  Port=2
  Dot Product : DotProduct  OutDataTypeStr=Inherit: Inherit via internal rule
  Earth's Radius : Constant  Value=env.Earth.R
  Eclipse (1) : Subsystem  TreatAsAtomicUnit=on
  Gain : Gain  Gain=-1
  If : If  NumInputs=2  IfExpression=u1 < u2
  Merge : Merge
  Norm : Subsystem
  NotEclipse (0) : Subsystem  TreatAsAtomicUnit=on
  Sqrt : Sqrt
  Square : Math  Operator=square
  Square1 : Math  Operator=square
  Subtract : Sum  Inputs=+-
  eclipseFlag : Outport
  wires:
  r_n/1 -> Dot Product/2, Norm/1(Vector)  "r_n"
  S_n/1 -> Dot Product/1  "S_n"
  Norm/1(Norm) -> Square1/1  "norm_r"
  If/1 -> Eclipse (1)/Action
  If/2 -> NotEclipse (0)/Action
  Merge/1 -> eclipseFlag/1
  Eclipse (1)/1(One) -> Merge/1
  NotEclipse (0)/1(Zero) -> Merge/2
  Dot Product/1 -> If/1
  Gain/1 -> If/2
  Sqrt/1 -> Gain/1
  Subtract/1 -> Sqrt/1
  Square/1 -> Subtract/2
  Square1/1 -> Subtract/1
  Earth's Radius/1 -> Square/1  "earth_R"

== system CubeSat/Real World/DKE (Dynamics Kinematics Environment)/Environment/Perturbations ==
  note: Gravity Gradiente
      | Solar Pressure
      | Magnetic torquer
      | Air drag ??
  S_n : Inport
  r_n : Inport  Port=2
  A_bn : Inport  Port=3
  A_bl : Inport  Port=4
  Constant : Constant  Value=[0; 0; 0]
  Gravity Gradient Torque : Subsystem
  Magnetic Field Torque : Subsystem
  MatrixMultiply : Product  Multiplication=Matrix(*)
  Solar Radiation Pressure Torque : Subsystem
  Sum : Sum  Inputs=++++
  Disturbance_torque : Outport
  wires:
  Sum/1 -> Disturbance_torque/1
  Solar Radiation Pressure Torque/1(T_srp) -> Sum/2
  S_n/1 -> MatrixMultiply/2
  A_bl/1 -> Gravity Gradient Torque/1(A_bl)
  r_n/1 -> Magnetic Field Torque/1(r_n), Gravity Gradient Torque/2(r_n)
  Gravity Gradient Torque/1(T_gg) -> Sum/1
  A_bn/1 -> MatrixMultiply/1, Magnetic Field Torque/2(A(B/N))
  Magnetic Field Torque/1(T_mag) -> Sum/3
  Constant/1 -> Sum/4
  MatrixMultiply/1 -> Solar Radiation Pressure Torque/1(S_b)  "S_b"

== system CubeSat/Real World/DKE (Dynamics Kinematics Environment)/Environment/Sun Direction Circular Orbit ==
  note: Input Interface
  note: Output Interface
  Clock : Clock
  Cos : Trigonometry  Operator=cos
  Cos1 : Trigonometry  Operator=cos
  Earth's Inclination : Constant  Value=env.Earth.i
  Gain : Gain  Gain=env.Earth.n
  Matrix Concatenate : Concatenate  NumInputs=3  Mode=Multidimensional array
  Product : Product
  Product1 : Product
  Product2 : Product
  Sin : Trigonometry
  Sin1 : Trigonometry
  Sun's Radius : Constant  Value=env.Sun.R
  S_n : Outport
  wires:
  Clock/1 -> Gain/1
  Gain/1 -> Sin/1, Cos/1
  Product/1 -> S_n/1
  Sun's Radius/1 -> Product/2
  Matrix Concatenate/1 -> Product/1
  Earth's Inclination/1 -> Sin1/1, Cos1/1
  Cos1/1 -> [cos]
  Sin1/1 -> [sin]
  Cos/1 -> Matrix Concatenate/1
  Product1/1 -> Matrix Concatenate/2
  Product2/1 -> Matrix Concatenate/3
  [sin] -> Product2/2
  [cos] -> Product1/1
  Sin/1 -> Product1/2, Product2/1

== system CubeSat/Real World/DKE (Dynamics Kinematics Environment)/Kinematics/Attitude Error ==
  A_bn : Inport
  A_ln : Inport  Port=2
  Matrix Multiply : Product  Multiplication=Matrix(*)
  Transpose : Math  Operator=transpose
  A_bl : Outport
  wires:
  Transpose/1 -> Matrix Multiply/2
  A_ln/1 -> Transpose/1
  Matrix Multiply/1 -> A_bl/1
  A_bn/1 -> Matrix Multiply/1

== system CubeSat/Real World/DKE (Dynamics Kinematics Environment)/Kinematics/EulerKinematicsdelay ==
  note: Logic
  note: The flag is set to -1 when 313 is used and to 1 when 312 is used
  w_b : Inport
  312 Propagator : Subsystem
  312To313 : Subsystem
  313 Propagator : Subsystem
  313To312 : Subsystem
  A312 : Subsystem
  A313 : Subsystem
  Abs : Abs  SaturateOnIntegerOverflow=off
  Cos : Trigonometry  Operator=cos
  IC : InitialCondition  Value=IC.angles
  IC1 : InitialCondition  Value=IC.angles
  IC3 : InitialCondition
  Relay : Relay  OnSwitchValue=0.75  OffSwitchValue=0.35  OffOutputValue=-1
  Selector1 : Selector  InputPortWidth=3  IndexOptions=Index vector (dialog)  Indices=[2]  OutputSizes=1
  Switch : Switch  Criteria=u2 > Threshold  SaturateOnIntegerOverflow=off  InputSameDT=off
  Switch1 : Switch  Criteria=u2 > Threshold  SaturateOnIntegerOverflow=off  InputSameDT=off
  To Workspace : ToWorkspace  VariableName=flag1  SampleTime=-1
  To Workspace1 : ToWorkspace  VariableName=eu312  SampleTime=-1
  To Workspace2 : ToWorkspace  VariableName=eu313  SampleTime=-1
  A_bn : Outport
  wires:
  Cos/1 -> Abs/1
  Selector1/1 -> Cos/1
  Abs/1 -> Relay/1
  A313/1(Out1) -> Switch/3
  w_b/1 -> 313 Propagator/2(w_b), 312 Propagator/2(w_b)  "w_b"
  313 Propagator/1(EA) -> [Euler313], A313/1(Euler Angles)  "EulerAngles313"
  A312/1(DCM) -> Switch/1
  Switch1/1 -> Selector1/1
  Switch/1 -> A_bn/1  "DCM"
  313To312/1(Out1) -> IC1/1
  312To313/1(Out1) -> IC/1
  IC1/1 -> 312 Propagator/1(IC)
  IC/1 -> 313 Propagator/3(IC)
  [EulerFlag] -> Switch/2, 312 Propagator/3(Reset), 313 Propagator/1(Reset)
  312 Propagator/1(EA) -> [Euler312], A312/1(Euler Angles)  "EulerAngles312"
  312 Propagator/2(Out1) -> 312To313/1(In1)
  313 Propagator/2(Out1) -> 313To312/1(In1)
  Relay/1 -> IC3/1
  [Euler312] -> To Workspace1/1, Switch1/1
  [Euler313] -> To Workspace2/1, Switch1/3
  [EulerFlag] -> Switch1/2
  IC3/1 -> To Workspace/1, [EulerFlag]

== system CubeSat/Real World/DKE (Dynamics Kinematics Environment)/Kinematics/Kepler Integrator1 ==
  Add : Sum  Inputs=+-
  Add1 : Sum
  Constant : Constant  Value=IC.theta
  Constant1 : Constant  Value=3/2
  Constant2 : Constant
  Constant3 : Constant  Value=2
  Constant4 : Constant  Value=orb.e
  Constant5 : Constant  Value=2
  Constant6 : Constant
  Cosh : Trigonometry  Operator=cos
  Divide : Product  Inputs=*/
  Gain : Gain  Gain=orb.n
  Gain1 : Gain  Gain=orb.e
  Integrator : Integrator  InitialConditionSource=external  WrapState=on  WrappedStateUpperValue=2*pi  WrappedStateLowerValue=0
  Power : Math  Operator=pow
  Power1 : Math  Operator=pow
  Power2 : Math  Operator=pow
  th : Outport
  wires:
  Constant/1 -> Integrator/2
  Integrator/1 -> Cosh/1, th/1
  Divide/1 -> Integrator/1
  Power/1 -> Divide/2
  Constant1/1 -> Power/2
  Constant2/1 -> Add/1
  Add/1 -> Power/1
  Power1/1 -> Add/2
  Constant3/1 -> Power1/2
  Constant4/1 -> Power1/1
  Gain/1 -> Divide/1
  Power2/1 -> Gain/1
  Constant5/1 -> Power2/2
  Add1/1 -> Power2/1
  Constant6/1 -> Add1/1
  Gain1/1 -> Add1/2
  Cosh/1 -> Gain1/1

== system CubeSat/Real World/DKE (Dynamics Kinematics Environment)/Kinematics/LVLH Evolution wtr of Earth ==
  th : Inport
  i : Inport  Port=2
  Constant1 : Constant
  Constant{2,4..10} (8 alike) : Constant  Value=0
  Constant3 : Constant
  Cos : Trigonometry  Operator=cos
  Cos1 : Trigonometry  Operator=cos
  Gain : Gain  Gain=-1
  Gain1 : Gain  Gain=-1
  Matrix Concatenate{,1..2,4..6} (6 alike) : Concatenate  NumInputs=3  Mode=Multidimensional array
  Matrix Concatenate3 : Concatenate  NumInputs=3  Mode=Multidimensional array  ConcatenateDimension=2
  Matrix Concatenate7 : Concatenate  NumInputs=3  Mode=Multidimensional array  ConcatenateDimension=2
  Matrix Multiply : Product  Multiplication=Matrix(*)
  Sin : Trigonometry
  Sin1 : Trigonometry
  A_ln : Outport
  wires:
  Cos/1 -> [cos]
  Matrix Concatenate1/1 -> Matrix Concatenate3/3
  th/1 -> Cos/1, Sin/1
  Matrix Concatenate/1 -> Matrix Concatenate3/1
  Constant5/1 -> Matrix Concatenate1/1
  Constant3/1 -> Matrix Concatenate1/3
  [cos] -> Matrix Concatenate/1
  Sin/1 -> [sin]
  Constant6/1 -> Matrix Concatenate2/3
  Constant7/1 -> Matrix Concatenate/3
  Constant4/1 -> Matrix Concatenate1/2
  Matrix Concatenate2/1 -> Matrix Concatenate3/2
  [cos] -> Matrix Concatenate2/2
  [sin] -> Matrix Concatenate2/1
  Gain/1 -> Matrix Concatenate/2
  [sin] -> Gain/1
  Cos1/1 -> [cosi]
  Sin1/1 -> [sini]
  i/1 -> Cos1/1, Sin1/1
  Matrix Multiply/1 -> A_ln/1
  Matrix Concatenate3/1 -> Matrix Multiply/1
  Matrix Concatenate7/1 -> Matrix Multiply/2
  Matrix Concatenate6/1 -> Matrix Concatenate7/2
  Matrix Concatenate5/1 -> Matrix Concatenate7/3
  Matrix Concatenate4/1 -> Matrix Concatenate7/1
  Constant1/1 -> Matrix Concatenate4/1
  Constant2/1 -> Matrix Concatenate4/2
  Constant8/1 -> Matrix Concatenate4/3
  Constant9/1 -> Matrix Concatenate6/1
  Constant10/1 -> Matrix Concatenate5/1
  [cosi] -> Matrix Concatenate5/3
  [cosi] -> Matrix Concatenate6/2
  [sini] -> Matrix Concatenate5/2
  [sini] -> Gain1/1
  Gain1/1 -> Matrix Concatenate6/3

== system CubeSat/Real World/DKE (Dynamics Kinematics Environment)/Kinematics/SpaceCraft position wrt ECI ==
  th : Inport
  Add : Sum
  Add1 : Sum  Inputs=+-
  Constant : Constant  Value=orb.i
  Constant1 : Constant  Value=orb.i
  Constant2 : Constant
  Constant3 : Constant
  Constant4 : Constant  Value=2
  Constant5 : Constant  Value=orb.e
  Cos : Trigonometry  Operator=cos
  Cos1 : Trigonometry  Operator=cos
  Cos2 : Trigonometry  Operator=cos
  Divide : Product  Inputs=*/
  Gain : Gain  Gain=orb.e
  Gain1 : Gain  Gain=orb.a
  Matrix Concatenate : Concatenate  NumInputs=3  Mode=Multidimensional array
  Power : Math  Operator=pow
  Product : Product
  Product1 : Product
  Product2 : Product
  Sin : Trigonometry
  Sin1 : Trigonometry
  r_n : Outport
  wires:
  Constant/1 -> Sin/1
  Cos1/1 -> Matrix Concatenate/1
  th/1 -> Sin1/1, Cos2/1, Cos1/1
  Product1/1 -> Matrix Concatenate/2
  Product/1 -> Matrix Concatenate/3
  Sin1/1 -> Product1/2, Product/1
  Sin/1 -> Product/2
  Constant1/1 -> Cos/1
  Cos/1 -> Product1/1
  Product2/1 -> r_n/1
  Matrix Concatenate/1 -> Product2/1
  Divide/1 -> Product2/2
  Constant2/1 -> Add/1
  Add/1 -> Divide/2
  Cos2/1 -> Gain/1
  Gain/1 -> Add/2
  Constant3/1 -> Add1/1
  Power/1 -> Add1/2
  Constant4/1 -> Power/2
  Constant5/1 -> Power/1
  Add1/1 -> Gain1/1
  Gain1/1 -> Divide/1

== system CubeSat/Real World/Hardware Models/Actuators/CMG + Control Logic ==
  In1 : Inport
  w_mesured : Inport  Port=2
  w : Inport  Port=3
  A assembler : Subsystem
  Add : Sum
  B assembler : Subsystem
  CMG : Subsystem
  Constant3 : Constant  Value=40
  Cross Product : matrix_library/Cross Product
  Degrees to Radians : simulink_extras/Transformations/Degrees to Radians
  Gain : Gain  Gain=-1
  MATLAB Function : MATLAB Function  TreatAsAtomicUnit=on
  Matrix Multiply : Product  Multiplication=Matrix(*)
  hr : Constant  Value=[1;1;1;1]  VectorParams1D=off
  Mc : Outport
  wires:
  B assembler/1(B) -> MATLAB Function/1(A)
  In1/1 -> Add/1
  CMG/2(Mc) -> Mc/1
  w_mesured/1 -> Cross Product/1
  w/1 -> CMG/2(w)
  Degrees to Radians/1 -> B assembler/1(beta), A assembler/2(beta)
  CMG/1(delta) -> A assembler/1(delta), B assembler/2(delta)
  Matrix Multiply/1 -> Cross Product/2
  Cross Product/1 -> Add/2
  A assembler/1(A) -> Matrix Multiply/1
  hr/1 -> Matrix Multiply/2
  Add/1 -> MATLAB Function/2(B)
  MATLAB Function/1(y) -> Gain/1
  Constant3/1 -> Degrees to Radians/1
  Gain/1 -> CMG/1(delta_dot)

== system CubeSat/Real World/Hardware Models/Sensors/MAGNETOMETER ==
  note: Missing errors:
      | -SCALE FACTORS ERROR, we can add it to have a more refined model
  B_b : Inport
  Add : Sum
  Cast To Single : DataTypeConversion  OutDataTypeStr=single  SaturateOnIntegerOverflow=off  RndMeth=Floor
  Constant : Constant  Value=sens.mag.flag
  Constant1 : Constant  Value=sens.mag.A_nonorth
  Constant3 : Constant  Value=sens.mag.A_mis
  Demux1 : Demux  Outputs=3
  Matrix Multiply : Product  Multiplication=Matrix(*)
  MatrixMultiply : Product  Multiplication=Matrix(*)
  Mux1 : Mux  Inputs=3
  Noise x : Subsystem
  Noise y : Subsystem
  Noise z : Subsystem
  Switch : Switch  Criteria=u2 > Threshold  SaturateOnIntegerOverflow=off  InputSameDT=off
  "discretization " : ZeroOrderHold  SampleTime=sens.mag.Ts
  quantization : Quantizer  QuantizationInterval=sens.mag.Quant
  saruration : Saturate  UpperLimit=sens.mag.sat(1,1)  LowerLimit=sens.mag.sat(1,2)
  B_meas_b : Outport
  wires:
  [B] -> Switch/3
  Constant/1 -> Switch/2
  Switch/1 -> quantization/1
  "discretization "/1 -> Cast To Single/1
  saruration/1 -> "discretization "/1
  quantization/1 -> saruration/1
  Constant3/1 -> Matrix Multiply/1
  Matrix Multiply/1 -> MatrixMultiply/2
  Constant1/1 -> MatrixMultiply/1
  MatrixMultiply/1 -> Add/1
  Cast To Single/1 -> B_meas_b/1
  Add/1 -> Switch/1
  Demux1/3 -> Noise z/1(Bz_real)
  B_b/1 -> Demux1/1, Matrix Multiply/2, [B]
  Demux1/1 -> Noise x/1(Bx_real)
  Noise x/1(Out1) -> Mux1/1
  Noise z/1(Out1) -> Mux1/3
  Noise y/1(Out1) -> Mux1/2
  Mux1/1 -> Add/2
  Demux1/2 -> Noise y/1(By_real)

== system CubeSat/Real World/Hardware Models/Sensors/SS Selector ==
  note: Take care of selecting which Sun Sensor is
      | seeing the sun at a given moment, prioritising the
      | Fine Sensor on the Top panel
      |
      | TODO :
      | Add a variable to switch weights in Wahba's Problem formulation if Fine Sensor is used
      |
      | Change Log
      | Created 18/12/2024
  Fine SS : Inport
  Course SS 1 : Inport  Port=2
  Course SS 2 : Inport  Port=3
  Course SS 3 : Inport  Port=4
  Course SS 4 : Inport  Port=5
  Norm1 : Subsystem
  Norm2 : Subsystem
  Norm3 : Subsystem
  Norm4 : Subsystem
  Switch{,1..3} (4 alike) : Switch  Criteria=u2 ~= 0  SaturateOnIntegerOverflow=off  InputSameDT=off
  Terminator : Terminator
  S_meas_b : Outport
  wires:
  Fine SS/1 -> [Fine], Norm1/1(Vector)
  Course SS 1/1 -> [Co1], Norm2/1(Vector)
  Course SS 2/1 -> [Co2], Norm3/1(Vector)
  Course SS 3/1 -> [Co3], Norm4/1(Vector)
  Switch/1 -> S_meas_b/1
  Switch1/1 -> Switch/3
  Norm1/1(Norm) -> [FineN]  "norm_r"
  Norm2/1(Norm) -> [Co1N]  "norm_r"
  Norm3/1(Norm) -> [Co2N]  "norm_r"
  Norm4/1(Norm) -> [Co3N]  "norm_r"
  Course SS 4/1 -> Terminator/1, [Co4]  "norm_r"
  Switch2/1 -> Switch1/3
  Switch3/1 -> Switch2/3
  [Co4] -> Switch3/3
  [Fine] -> Switch/1
  [FineN] -> Switch/2
  [Co1] -> Switch1/1
  [Co1N] -> Switch1/2
  [Co2] -> Switch2/1
  [Co2N] -> Switch2/2
  [Co3] -> Switch3/1
  [Co3N] -> Switch3/2
